simulink model "TransmissionController"  (R2020b)
settings: Solver=VariableStepAuto  StartTime=0.0  StopTime=10.0  RelTol=1e-3
undefined symbols (not defined in the file): EMAP, Iei, Kfactor, NE_VEC, speedratio, TH_VEC, Torkratio
settings Model: Creator=priyaD  LastModifiedBy=priyaD

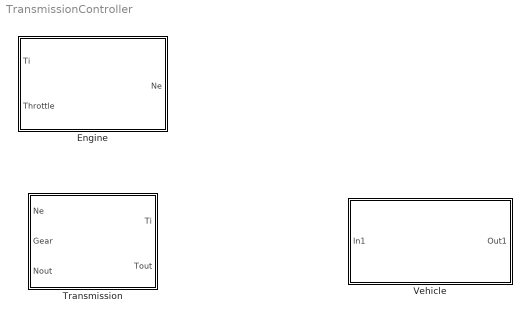
== system TransmissionController ==
  Engine : Subsystem
  Transmission : Subsystem
  Vehicle : Subsystem

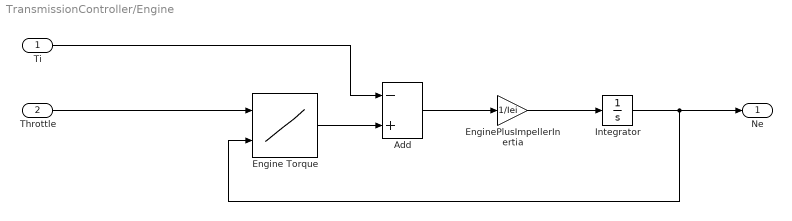
== system TransmissionController/Engine ==
  Ti : Inport
  Throttle : Inport  Port=2
  Add : Sum  Inputs=-+
  Engine Torque : Lookup_n-D  BreakpointsForDimension1=TH_VEC  BreakpointsForDimension2=NE_VEC  Table=EMAP  InputSameDT=on
      settings: InputPortMap=u0,u1
  EnginePlusImpellerInertia : Gain  Gain=1/Iei
  Integrator : Integrator  InitialCondition=1000  LimitOutput=on  UpperSaturationLimit=6000  LowerSaturationLimit=600  ZeroCross=off
  Ne : Outport
  wires:
  Ti/1 -> Add/1
  EnginePlusImpellerInertia/1 -> Integrator/1
  Throttle/1 -> Engine Torque/1
  Integrator/1 -> Ne/1, Engine Torque/2
  Add/1 -> EnginePlusImpellerInertia/1
  Engine Torque/1 -> Add/2

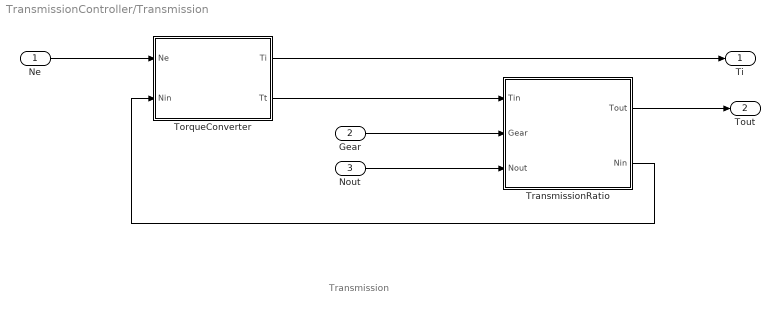
== system TransmissionController/Transmission ==
  note: Transmission
  Ne : Inport
  Gear : Inport  Port=2
  Nout : Inport  Port=3
  TorqueConverter : Subsystem
  TransmissionRatio : Subsystem
  Ti : Outport
  Tout : Outport  Port=2
  wires:
  Gear/1 -> TransmissionRatio/2(Gear)
  Nout/1 -> TransmissionRatio/3(Nout)
  TorqueConverter/2(Tt) -> TransmissionRatio/1(Tin)
  TransmissionRatio/2(Nin) -> TorqueConverter/2(Nin)
  TorqueConverter/1(Ti) -> Ti/1
  TransmissionRatio/1(Tout) -> Tout/1
  Ne/1 -> TorqueConverter/1(Ne)

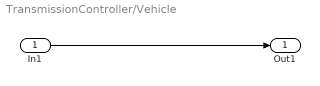
== system TransmissionController/Vehicle ==
  In1 : Inport
  Out1 : Outport
  wires:
  In1/1 -> Out1/1

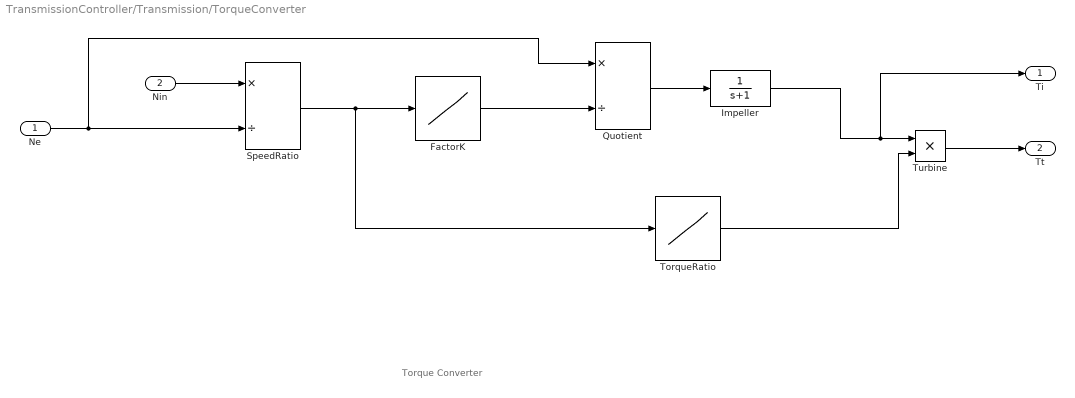
== system TransmissionController/Transmission/TorqueConverter ==
  note: Torque Converter
  Ne : Inport
  Nin : Inport  Port=2
  FactorK : Lookup_n-D  NumberOfTableDimensions=1  BreakpointsForDimension1=speedratio  Table=Kfactor  SaturateOnIntegerOverflow=on  InputSameDT=on
  Impeller : TransferFcn  Denominator=[1 1]
  Quotient : Product  Inputs=*/  SaturateOnIntegerOverflow=on
  SpeedRatio : Product  Inputs=*/  SaturateOnIntegerOverflow=on
  TorqueRatio : Lookup_n-D  NumberOfTableDimensions=1  BreakpointsForDimension1=speedratio  Table=Torkratio  SaturateOnIntegerOverflow=on  InputSameDT=on
  Turbine : Product  SaturateOnIntegerOverflow=on
  Ti : Outport
  Tt : Outport  Port=2
  wires:
  FactorK/1 -> Quotient/2
  Nin/1 -> SpeedRatio/1
  Turbine/1 -> Tt/1
  SpeedRatio/1 -> TorqueRatio/1, FactorK/1
  TorqueRatio/1 -> Turbine/2
  Impeller/1 -> Ti/1, Turbine/1
  Ne/1 -> Quotient/1, SpeedRatio/2
  Quotient/1 -> Impeller/1

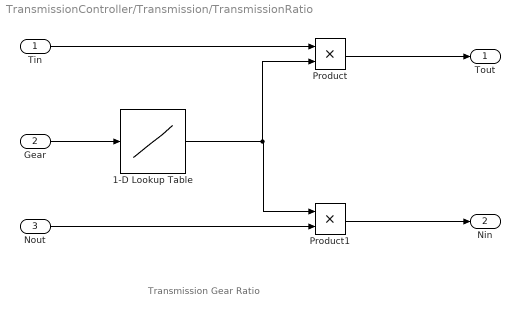
== system TransmissionController/Transmission/TransmissionRatio ==
  note: Transmission Gear Ratio
  Tin : Inport
  Gear : Inport  Port=2
  Nout : Inport  Port=3
  1-D Lookup Table : Lookup_n-D  NumberOfTableDimensions=1  BreakpointsForDimension1=[1 2 3 4]  Table=[2.393 1.450 1.000 0.677]  SaturateOnIntegerOverflow=on  InputSameDT=on
  Product : Product  SaturateOnIntegerOverflow=on
  Product1 : Product  SaturateOnIntegerOverflow=on
  Tout : Outport
  Nin : Outport  Port=2
  wires:
  Product1/1 -> Nin/1
  Nout/1 -> Product1/2
  Gear/1 -> 1-D Lookup Table/1
  1-D Lookup Table/1 -> Product/2, Product1/1
  Tin/1 -> Product/1
  Product/1 -> Tout/1
